simulink model "automata_learning"  (R2022a)
settings: Solver=FixedStepAuto  StartTime=0.0  StopTime=10.0  FixedStep=0.005  RelTol=1e-3
(part 1 of 14)
settings Model: Creator=diego  LastModifiedBy=diego

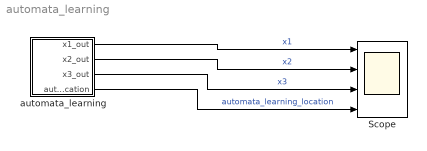
== system automata_learning ==
  Scope : Scope  NumInputPorts=4
  automata_learning : Stateflow chart  TreatAsAtomicUnit=on
  wires:
  automata_learning/1(x1_out) -> Scope/1  "x1"
  automata_learning/2(x2_out) -> Scope/2  "x2"
  automata_learning/3(x3_out) -> Scope/3  "x3"
  automata_learning/4(automata_learning_location) -> Scope/4  "automata_learning_location"
